simulink model "SpectrumAnalyzerMeasurementsExample"  (R2014a)
settings: Solver=FixedStepDiscrete  StartTime=0.0  StopTime=Inf  RelTol=1e-3
libraries: dspsrcs4 x13, dsppolyfun x5, dspmlti4 x2, dspmisc x1
settings Model: Creator=The MathWorks Inc.
settings SFSimCC: SimGenImportedTypeDefs=on

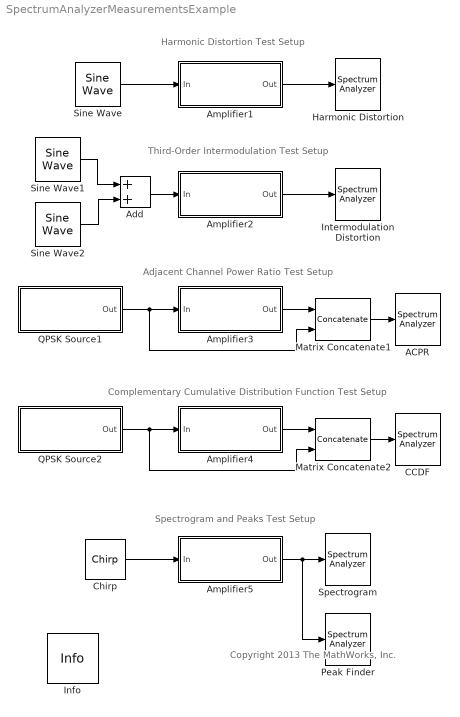
== system SpectrumAnalyzerMeasurementsExample ==
  note: Spectrogram and Peaks Test Setup
  note: Adjacent Channel Power Ratio Test Setup
  note: Third-Order Intermodulation Test Setup
  note: Harmonic Distortion Test Setup
  note: Complementary Cumulative Distribution Function Test Setup
  note: Copyright 2013 The MathWorks, Inc.
  ACPR : SpectrumAnalyzer
  Add : Sum
  Amplifier1 : Subsystem  TreatAsAtomicUnit=on
  Amplifier2 : Subsystem  TreatAsAtomicUnit=on
  Amplifier3 : Subsystem  TreatAsAtomicUnit=on
  Amplifier4 : Subsystem  TreatAsAtomicUnit=on
  Amplifier5 : Subsystem  TreatAsAtomicUnit=on
  CCDF : SpectrumAnalyzer
  Chirp : dspsrcs4/Chirp  sweep=Quadratic  mode=Bidirectional  f0=2.5e6  f1=5e6  t1=1e-3  Tsweep=1e-3  phase=0  Ts=1/10/3.84e6  spf=10  datatype=Double
  Harmonic Distortion : SpectrumAnalyzer
  Info : dspmisc/Info  SystemSampleTime=-1
  Intermodulation Distortion : SpectrumAnalyzer
  Matrix Concatenate1 : Concatenate  Mode=Multidimensional array  ConcatenateDimension=2
  Matrix Concatenate2 : Concatenate  Mode=Multidimensional array  ConcatenateDimension=2
  Peak Finder : SpectrumAnalyzer
  QPSK Source1 : Subsystem  TreatAsAtomicUnit=on
  QPSK Source2 : Subsystem  TreatAsAtomicUnit=on
  Sine Wave : dspsrcs4/Sine Wave  Amplitude=1  Frequency=2e6  Phase=0  SampleMode=Discrete  OutComplex=Real  CompMethod=Trigonometric fcn  TableSize=Speed  SampleTime=1/10/3.84e6  SamplesPerFrame=10  ResetState=Restart at time zero  dataType=double  wordLen=16  udDataType=sfix(16)  fracBitsMode=Best precision  numFracBits=15  OutDataTypeStr=double  LastOutDataTypeStr=double
  Sine Wave1 : dspsrcs4/Sine Wave  Amplitude=1  Frequency=9e6  Phase=0  SampleMode=Discrete  OutComplex=Real  CompMethod=Trigonometric fcn  TableSize=Speed  SampleTime=1/10/3.84e6  SamplesPerFrame=10  ResetState=Restart at time zero  dataType=double  wordLen=16  udDataType=sfix(16)  fracBitsMode=Best precision  numFracBits=15  OutDataTypeStr=double  LastOutDataTypeStr=double
  Sine Wave2 : dspsrcs4/Sine Wave  Amplitude=1  Frequency=11e6  Phase=0  SampleMode=Discrete  OutComplex=Real  CompMethod=Trigonometric fcn  TableSize=Speed  SampleTime=1/10/3.84e6  SamplesPerFrame=10  ResetState=Restart at time zero  dataType=double  wordLen=16  udDataType=sfix(16)  fracBitsMode=Best precision  numFracBits=15  OutDataTypeStr=double  LastOutDataTypeStr=double
  Spectrogram : SpectrumAnalyzer
  wires:
  Amplifier1/1(Out) -> Harmonic Distortion/1
  Sine Wave/1 -> Amplifier1/1(In)
  Sine Wave1/1 -> Add/1
  Sine Wave2/1 -> Add/2
  Add/1 -> Amplifier2/1(In)
  Amplifier2/1(Out) -> Intermodulation Distortion/1
  QPSK Source1/1(Out) -> Matrix Concatenate1/2, Amplifier3/1(In)
  Matrix Concatenate1/1 -> ACPR/1
  Amplifier3/1(Out) -> Matrix Concatenate1/1
  Chirp/1 -> Amplifier5/1(In)
  Amplifier5/1(Out) -> Peak Finder/1, Spectrogram/1
  QPSK Source2/1(Out) -> Matrix Concatenate2/2, Amplifier4/1(In)
  Matrix Concatenate2/1 -> CCDF/1
  Amplifier4/1(Out) -> Matrix Concatenate2/1

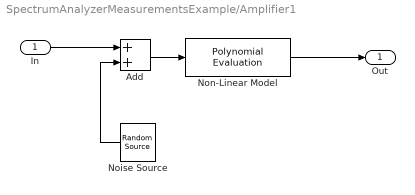
== system SpectrumAnalyzerMeasurementsExample/Amplifier1 ==
  In : Inport
  Add : Sum
  Noise Source : dspsrcs4/Random Source  SrcType=Gaussian  NormMethod=Ziggurat  CltLength=12  MinVal=0  MaxVal=1  MeanVal=0  VarVal=4e-16  RepMode=Not repeatable  rawSeed=1  IsInherit=off  SampMode=Discrete  SampTime=1/10/3.84e6  SampFrame=10  DataType=Double  OutComplex=Real
  Non-Linear Model : dsppolyfun/Polynomial Evaluation  useConstCoeffs=on  constCoeffs=[1e-6 1e-9 1e-5 1e-9 1e-6 5e-8 .5e-3 1e-6 1 3e-3]
  Out : Outport
  wires:
  Non-Linear Model/1 -> Out/1
  In/1 -> Add/1
  Add/1 -> Non-Linear Model/1
  Noise Source/1 -> Add/2

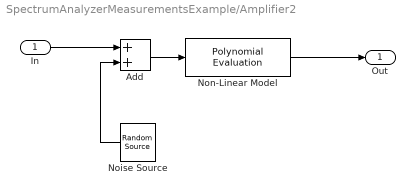
== system SpectrumAnalyzerMeasurementsExample/Amplifier2 ==
  In : Inport
  Add : Sum
  Noise Source : dspsrcs4/Random Source  SrcType=Gaussian  NormMethod=Ziggurat  CltLength=12  MinVal=0  MaxVal=1  MeanVal=0  VarVal=4e-14  RepMode=Not repeatable  rawSeed=1  IsInherit=off  SampMode=Discrete  SampTime=1/10/3.84e6  SampFrame=10  DataType=Double  OutComplex=Real
  Non-Linear Model : dsppolyfun/Polynomial Evaluation  useConstCoeffs=on  constCoeffs=[1e-6 1e-9 1e-5 1e-9 1e-6 5e-8 .5e-3 1e-6 1 3e-3]
  Out : Outport
  wires:
  Non-Linear Model/1 -> Out/1
  In/1 -> Add/1
  Add/1 -> Non-Linear Model/1
  Noise Source/1 -> Add/2

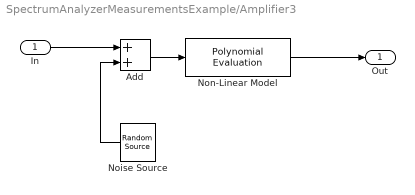
== system SpectrumAnalyzerMeasurementsExample/Amplifier3 ==
  In : Inport
  Add : Sum
  Noise Source : dspsrcs4/Random Source  SrcType=Gaussian  NormMethod=Ziggurat  CltLength=12  MinVal=0  MaxVal=1  MeanVal=0  VarVal=4e-14  RepMode=Not repeatable  rawSeed=1  IsInherit=off  SampMode=Discrete  SampTime=1/10/3.84e6  SampFrame=10  DataType=Double  OutComplex=Real
  Non-Linear Model : dsppolyfun/Polynomial Evaluation  useConstCoeffs=on  constCoeffs=[1e-6 1e-9 1e-5 1e-9 1e-6 5e-8 .5e-3 1e-6 1 3e-3]
  Out : Outport
  wires:
  Non-Linear Model/1 -> Out/1
  In/1 -> Add/1
  Add/1 -> Non-Linear Model/1
  Noise Source/1 -> Add/2

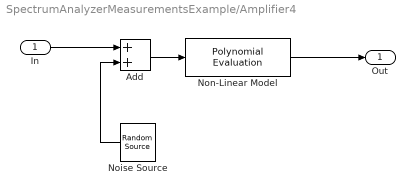
== system SpectrumAnalyzerMeasurementsExample/Amplifier4 ==
  In : Inport
  Add : Sum
  Noise Source : dspsrcs4/Random Source  SrcType=Gaussian  NormMethod=Ziggurat  CltLength=12  MinVal=0  MaxVal=1  MeanVal=0  VarVal=4e-14  RepMode=Not repeatable  rawSeed=1  IsInherit=off  SampMode=Discrete  SampTime=1/10/3.84e6  SampFrame=10  DataType=Double  OutComplex=Real
  Non-Linear Model : dsppolyfun/Polynomial Evaluation  useConstCoeffs=on  constCoeffs=[-1e-6 1e-9 -1e-5 1e-9 -1e-6 5e-8 -.5e-3 1e-6 1 3e-3]
  Out : Outport
  wires:
  Non-Linear Model/1 -> Out/1
  In/1 -> Add/1
  Add/1 -> Non-Linear Model/1
  Noise Source/1 -> Add/2

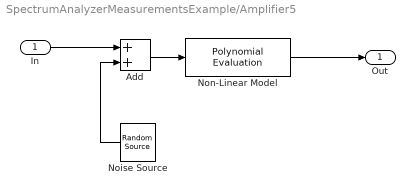
== system SpectrumAnalyzerMeasurementsExample/Amplifier5 ==
  In : Inport
  Add : Sum
  Noise Source : dspsrcs4/Random Source  SrcType=Gaussian  NormMethod=Ziggurat  CltLength=12  MinVal=0  MaxVal=1  MeanVal=0  VarVal=4e-14  RepMode=Not repeatable  rawSeed=1  IsInherit=off  SampMode=Discrete  SampTime=1/10/3.84e6  SampFrame=10  DataType=Double  OutComplex=Real
  Non-Linear Model : dsppolyfun/Polynomial Evaluation  useConstCoeffs=on  constCoeffs=[1e-6 1e-9 1e-5 1e-9 1e-6 5e-8 .5e-3 1e-6 1 3e-3]
  Out : Outport
  wires:
  Non-Linear Model/1 -> Out/1
  In/1 -> Add/1
  Add/1 -> Non-Linear Model/1
  Noise Source/1 -> Add/2

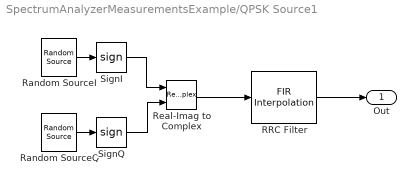
== system SpectrumAnalyzerMeasurementsExample/QPSK Source1 ==
  RRC Filter : dspmlti4/FIR Interpolation  h=5*rcosdesign(0.5, 20, 10, 'sqrt')  L=10  framing=Enforce single-rate processing  outputBufInitCond=0  InputProcessing=Columns as channels (frame based)  firstCoeffDataTypeStr=Inherit: Same word length as input  firstCoeffLastDataTypeStr=Inherit: Same word length as input  firstCoeffMin=[]  firstCoeffMax=[]  outputDataTypeStr=Inherit: Same as accumulator  outputLastDataTypeStr=Inherit: Same as accumulator  outputMin=[]  outputMax=[]  roundingMode=Floor  overflowMode=off  FilterSource=Specify via dialog  FilterObject=Hm_firinterp
  Random SourceI : dspsrcs4/Random Source  SrcType=Uniform  NormMethod=Ziggurat  CltLength=12  MinVal=-1  MaxVal=1  MeanVal=0  VarVal=1  RepMode=Not repeatable  rawSeed=1  IsInherit=off  SampMode=Discrete  SampTime=1/3.84e6  SampFrame=1  DataType=Double  OutComplex=Real
  Random SourceQ : dspsrcs4/Random Source  SrcType=Uniform  NormMethod=Ziggurat  CltLength=12  MinVal=-1  MaxVal=1  MeanVal=0  VarVal=1  RepMode=Not repeatable  rawSeed=1  IsInherit=off  SampMode=Discrete  SampTime=1/3.84e6  SampFrame=1  DataType=Double  OutComplex=Real
  Real-Imag to Complex : RealImagToComplex
  SignI : Signum
  SignQ : Signum
  Out : Outport
  wires:
  Random SourceI/1 -> SignI/1
  Random SourceQ/1 -> SignQ/1
  SignI/1 -> Real-Imag to Complex/1
  SignQ/1 -> Real-Imag to Complex/2
  Real-Imag to Complex/1 -> RRC Filter/1
  RRC Filter/1 -> Out/1

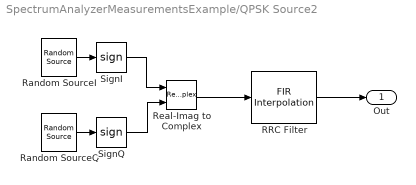
== system SpectrumAnalyzerMeasurementsExample/QPSK Source2 ==
  RRC Filter : dspmlti4/FIR Interpolation  h=6*rcosdesign(0.5, 20, 10, 'sqrt')  L=10  framing=Enforce single-rate processing  outputBufInitCond=0  InputProcessing=Columns as channels (frame based)  firstCoeffDataTypeStr=Inherit: Same word length as input  firstCoeffLastDataTypeStr=Inherit: Same word length as input  firstCoeffMin=[]  firstCoeffMax=[]  outputDataTypeStr=Inherit: Same as accumulator  outputLastDataTypeStr=Inherit: Same as accumulator  outputMin=[]  outputMax=[]  roundingMode=Floor  overflowMode=off  FilterSource=Specify via dialog  FilterObject=Hm_firinterp
  Random SourceI : dspsrcs4/Random Source  SrcType=Uniform  NormMethod=Ziggurat  CltLength=12  MinVal=-1  MaxVal=1  MeanVal=0  VarVal=1  RepMode=Not repeatable  rawSeed=1  IsInherit=off  SampMode=Discrete  SampTime=1/3.84e6  SampFrame=1  DataType=Double  OutComplex=Real
  Random SourceQ : dspsrcs4/Random Source  SrcType=Uniform  NormMethod=Ziggurat  CltLength=12  MinVal=-1  MaxVal=1  MeanVal=0  VarVal=1  RepMode=Not repeatable  rawSeed=1  IsInherit=off  SampMode=Discrete  SampTime=1/3.84e6  SampFrame=1  DataType=Double  OutComplex=Real
  Real-Imag to Complex : RealImagToComplex
  SignI : Signum
  SignQ : Signum
  Out : Outport
  wires:
  Random SourceI/1 -> SignI/1
  Random SourceQ/1 -> SignQ/1
  SignI/1 -> Real-Imag to Complex/1
  SignQ/1 -> Real-Imag to Complex/2
  Real-Imag to Complex/1 -> RRC Filter/1
  RRC Filter/1 -> Out/1
